simulink model "hw2_1_mdl"  (R2024b)
settings: Solver=ode4  StartTime=0.0  StopTime=simTime  FixedStep=sampling_time  RelTol=1e-3
values from neighbouring files (symbols this model uses):
  a = rand*10    [hw2_1.m]    (also in hw2_2.m)
  b = rand*10    [hw2_1.m]    (also in hw2_2.m)
  gamma = 1    [hw2_1.m]
  inputMagnitude = 1    [hw2_1.m]    (also in hw2_2.m = 10)
  sampling_time = 0.01    [hw2_1.m]    (also in hw2_2.m)
settings Model: Creator=kemal  LastModifiedBy=kemal

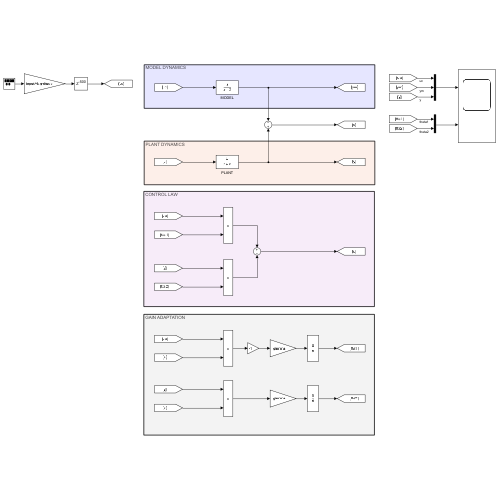
[thumbnail: Simulink's stored preview of the top-level diagram]
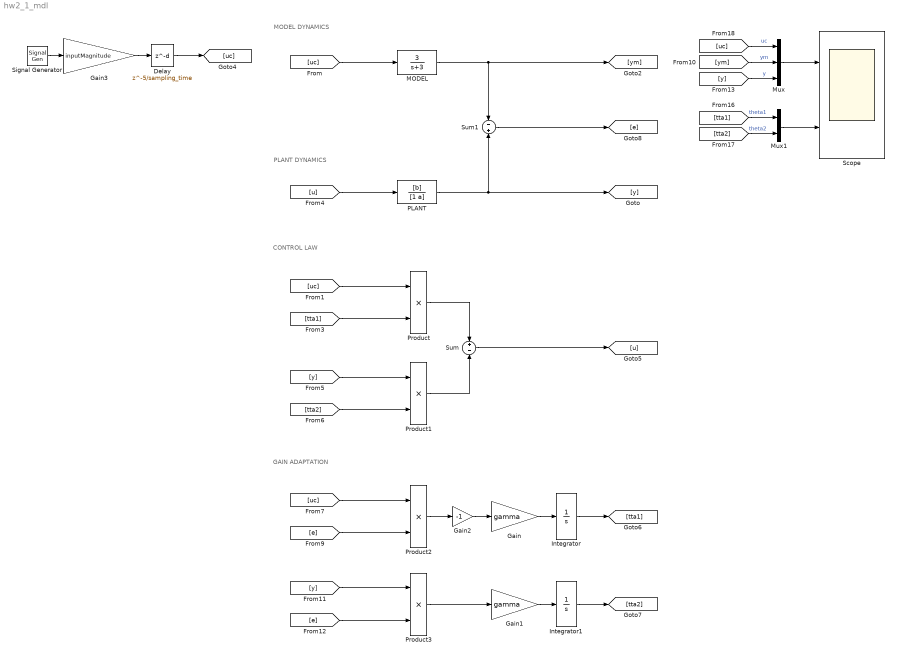
== system hw2_1_mdl ==
  note: GAIN ADAPTATION
  note: CONTROL LAW
  note: MODEL DYNAMICS
  note: PLANT DYNAMICS
  Delay : Delay  DelayLength=5/sampling_time
  Gain : Gain  Gain=gamma
  Gain1 : Gain  Gain=gamma
  Gain2 : Gain  Gain=-1
  Gain3 : Gain  Gain=inputMagnitude
  Integrator : Integrator
  Integrator1 : Integrator
  MODEL : TransferFcn  Numerator=3  Denominator=[1 3]
  Mux : Mux  Inputs=3
  Mux1 : Mux  Inputs=2
  PLANT : TransferFcn  Numerator=[b]  Denominator=[1 a]
  Product{,1..3} (4 alike) : Product
  Scope : Scope  NumInputPorts=2
  Signal Generator : SignalGenerator  WaveForm=square  Frequency=0.1
  Sum : Sum  Inputs=+-
  Sum1 : Sum  Inputs=-+
  wires:
  PLANT/1 -> Sum1/2, [y]
  MODEL/1 -> Sum1/1, [ym]
  [uc] -> MODEL/1
  [tta1] -> Product/2
  Product/1 -> Sum/1
  [tta2] -> Product1/2
  [y] -> Product1/1
  Product1/1 -> Sum/2
  Sum/1 -> [u]
  Signal Generator/1 -> Gain3/1
  [u] -> PLANT/1
  Integrator/1 -> [tta1]
  Sum1/1 -> [e]
  [uc] -> Product2/1
  [e] -> Product2/2
  Product2/1 -> Gain2/1
  Gain/1 -> Integrator/1
  Gain1/1 -> Integrator1/1
  Product3/1 -> Gain1/1
  [e] -> Product3/2
  [y] -> Product3/1
  Integrator1/1 -> [tta2]
  Gain2/1 -> Gain/1
  [ym] -> Mux/2  "ym"
  [y] -> Mux/3  "y"
  Mux/1 -> Scope/1
  [tta1] -> Mux1/1  "theta1"
  [tta2] -> Mux1/2  "theta2"
  [uc] -> Mux/1  "uc"
  Delay/1 -> [uc]
  Gain3/1 -> Delay/1
  [uc] -> Product/1
  Mux1/1 -> Scope/2
